simulink model "TVModel_Simulation_21"  (R2021b)
settings: Solver=FixedStepDiscrete  StartTime=0.0  StopTime=250  FixedStep=0.02  MaxStep=0.01  RelTol=1e-3
undefined symbols (not defined in the file or in its folder): MB, TV, TV_OLD
libraries: simulink x22, simulink_extras x14, eeGeneralControl x13, slpidlib x8, fuzblock x4, controlLib x4, cstblocks x3, dspstat3 x2, eeSlidingModeController x1, sharedTrackingLibrary x1
(part 9 of 9)

== matlab function TVModel_Simulation_21/Subsystem/Subsystem1/Torque Distribution/MPC/     Output Vector Reference/MATLAB Function ==
  data: u input; y output
function y = fcn(u)

N = 2;
n = N-1;
y = repmat(u,n,1);

== matlab function TVModel_Simulation_21/Subsystem/Subsystem1/Torque Distribution/MPC/Mz Generation/MATLAB Function ==
  data: u input; Mzlb output; epsilon input; Mzub output
function [Mzlb,Mzub] = fcn(u,epsilon)

if epsilon == 0
   Mzlb = -0.1;
   Mzub = 0.1;
else
   Mzub = u;
   Mzlb = -u;
end

== matlab function TVModel_Simulation_21/Subsystem/Subsystem1/Torque Distribution/MPC/States Constraints/MATLAB Function ==
  data: u input; y output
function y = fcn(u)

N=2;
n = N-1;
y = repmat(u,n,1);

== matlab function TVModel_Simulation_21/Subsystem/Subsystem1/Torque Distribution/MPC/States Constraints/MATLAB Function1 ==
  data: u input; y output
function y = fcn(u)

N=2;
n = N-1;
y = repmat(u,n,1);

== stateflow chart TVModel_Simulation_21/Subsystem/Subsystem1/Slip Control/Traction Control/ABS/Subsystem/Chart1 ==
  state OFF
    en,du:
    TC_max = [21];
  state ON
    en,du:
    TC_max = T_ff ;
  state SWITCHING_FILTER
    en,du:
    TC_max = TC_filter_tau*TC_max;
  (default) -> OFF
  OFF -> ON : [epsilon == 1]
  SWITCHING_FILTER -> ON [order 2] : [ epsilon == 1]
  SWITCHING_FILTER -> OFF [order 1] : [count(in(SWITCHING_FILTER)) > TC_filter_time/ts]
  ON -> SWITCHING_FILTER : [epsilon == 0]
  data: T_ff input; TC_max output; ts constant double =TV.MPC.T; TC_filter_time constant double =TV.MPC.mz_filter_time; TC_filter_tau constant double =TV.MPC.mz_filter_tau; epsilon input

== matlab function TVModel_Simulation_21/Subsystem/Subsystem1/Torque Distribution/MPC/Control Constraints/MATLAB Function1 ==
  data: u input; y output; N input
function y = fcn(u,N)

% n = N;
% y = zeros(n*length(u));
n = 2;
y = repmat(u,n,1);

== matlab function TVModel_Simulation_21/Subsystem/Subsystem1/Torque Distribution/MPC/Polytopic Constraints/Driver Inputs/MATLAB Function3 ==
  data: lbx input; lg_saturation output
function lg_saturation = fcn(lbx)

max_front = max(lbx(1),lbx(2));
max_rear  = max(lbx(3),lbx(4));

lg_saturation = 2*(max_front+max_rear);

== matlab function TVModel_Simulation_21/Subsystem/Subsystem1/Torque Distribution/MPC/Polytopic Constraints/Driver Inputs/MATLAB Function4 ==
  data: ubx input; ug_saturation output
function ug_saturation = fcn(ubx)

min_front = min(ubx(1),ubx(2));
min_rear  = min(ubx(3),ubx(4));

ug_saturation = 2*(min_front+min_rear);

== stateflow chart TVModel_Simulation_21/Subsystem/Subsystem1/Slip Control/Traction Control/ABS/Subsystem/Chart2 ==
  state OFF
    en,du:
    TC_max = [21];
  state ON
    en,du:
    TC_max = T_ff ;
  state SWITCHING_FILTER
    en,du:
    TC_max = TC_filter_tau*TC_max;
  (default) -> OFF
  OFF -> ON : [epsilon == 1]
  SWITCHING_FILTER -> ON [order 2] : [ epsilon == 1]
  SWITCHING_FILTER -> OFF [order 1] : [count(in(SWITCHING_FILTER)) > TC_filter_time/ts]
  ON -> SWITCHING_FILTER : [epsilon == 0]
  data: T_ff input; TC_max output; ts constant double =TV.MPC.T; TC_filter_time constant double =TV.MPC.mz_filter_time; TC_filter_tau constant double =TV.MPC.mz_filter_tau; epsilon input

== stateflow chart TVModel_Simulation_21/Subsystem/Subsystem1/Slip Control/Traction Control/ABS/Subsystem/Chart3 ==
  state OFF
    en,du:
    TC_max = [21];
  state ON
    en,du:
    TC_max = T_ff ;
  state SWITCHING_FILTER
    en,du:
    TC_max = TC_filter_tau*TC_max;
  (default) -> OFF
  OFF -> ON : [epsilon == 1]
  SWITCHING_FILTER -> ON [order 2] : [ epsilon == 1]
  SWITCHING_FILTER -> OFF [order 1] : [count(in(SWITCHING_FILTER)) > TC_filter_time/ts]
  ON -> SWITCHING_FILTER : [epsilon == 0]
  data: T_ff input; TC_max output; ts constant double =TV.MPC.T; TC_filter_time constant double =TV.MPC.mz_filter_time; TC_filter_tau constant double =TV.MPC.mz_filter_tau; epsilon input
